simulink model "test_com_SensorFusion_SF_D4_slip_GPS"  (R2019b)
settings: Solver=FixedStepDiscrete  StartTime=0  StopTime=stop  FixedStep=0.001  RelTol=1e-3
undefined symbols (not defined in the file or in its folder): BxTM, ByTM, CxTM, CyTM, g, gamma_stat_front, gamma_stat_rear, gearbox_ratio, l_F, l_R, m_sprung, m_unsprung_quarter, mag_calib_front_center, mag_calib_front_compmatrix, mag_calib_rear_center, mag_calib_rear_compmatrix, should_be_in_theSensorFusion, switch_VelYcalculation_pSF, testStart_VelX_pSF, testVelY_pSF, tire_r_dyn, track_angle_front, track_width_front, track_width_rear, v2o_x, wheel_kinematics_breakpoints, wheel_kinematics_FL_data, wheel_kinematics_FR_data, wheelbase, x9DFrontX, x9DFrontY, x9DRearX, x9DRearY
libraries: SignalProcessingSensorFusionLib x30, simulink x6
(part 8 of 9)

== matlab function test_com_SensorFusion_SF_D4_slip_GPS/Subsystem14/SensorFusion_D4/SF_LaKl_GPS ==
  data: x9DFront input Bus: control_9D; VehicleState output Bus: control_VehicleState; x9DRear input Bus: control_9D; v2o input Bus: control_Velocity; WheelSpeeds input; WheelSpeeds_Sq input; RockerAngle input; RockerAngle_Sq input; dt input; kalman_running output; tire_r_dyn parameter; GPS input
function [VehicleState,kalman_running]  = fcn(x9DFront, x9DRear, v2o, WheelSpeeds, WheelSpeeds_Sq, RockerAngle, RockerAngle_Sq, dt, tire_r_dyn, GPS)
%% SAE is the used KOS, global not local on the car -> trafo of measurements in global KOS necessary
persistent state P

persistent standstill_counter
persistent bias_measurements 
persistent P_bias

persistent YawAngle_Front_old YawAngle_Rear_old v2o_VelX_old


num_states= 7;
num_measurements=5;


% copied from E10 SF .. might work
YawAngle_measurement=single(0);
R_YawAngle=1000;


% state   =   (1) PosX
%             (2) PosY
%             (3) PosZ
%             (4) VelX
%             (5) VelY
%             (6) VelZ
%             (7) YawAngle
%             (8)YawRate
% %             (9)WheelVelocity_FL
% %             (10)WheelVelocity_FR
% %             (11)WheelVelocity_RL
% %             (12)WheelVelocity_RR
     

% Actually used measurements:
%               (1) VelX
%               (2) VelY
%               (3) AccX front
%               (4) AccY front
%               (5) AccZ front
%               (6) YawAngle_Front
%               (7) YawRate_Front
%               (8) wheelvelocity_FL
%               (9) wheelvelocity_FR
%               (10) wheelvelocity_RL
%               (11)wheelvelocity_RR



if isempty(P)
    
    P_bias=single(eye(num_measurements));%*0.01);
    standstill_counter=0;
    bias_measurements=single(zeros(num_measurements,1));
    

    state = single(zeros(num_states,1));
    P = single(eye(num_states, num_states));%*0.1);
    
    YawAngle_Front_old=single(0);
    YawAngle_Rear_old=single(0);
    v2o_VelX_old=single(0);
    
end




%% Readability

PosX=       state(1);
PosY=       state(2);
PosZ=       state(3);
VelX=       state(4);
VelY=       state(5);
VelZ=       state(6);
YawAngle=   state(7);
%YawRate=    state(8);
% Wheelvel_FL= state(9);
% Wheelvel_FR= state(10);
% Wheelvel_RL= state(11);
% Wheelvel_RR= state(12);

AccX = x9DFront.AccX;
AccY = x9DFront.AccY;
AccZ = x9DFront.AccZ;
YawRate = x9DFront.YawRate;
GPS_Long = (GPS.GPS_Longitude-8.5);%*100000;
GPS_Lat = (GPS.GPS_Latitude-49.30);%*100000;


    measurements= [
% v2o.VelX            % (1)   v2o Sensor x velocity
% v2o.VelY            % (2)   v2o Sensor y velocity
% v2o.SlipAngle       % (3)   v2o Sensor Slipangle
% x9DFront.AccX       % (4)   IMU Front  x acceleration
% x9DFront.AccY       % (5)   IMU Front  y acceleration
% x9DFront.AccZ       % (6)   IMU Front  z acceleration
% x9DFront.RollRate   % (7)   IMU Front  RollRate
% x9DFront.PitchRate  % (8)   IMU Front  PitchRate
% x9DFront.YawRate    % (9)   IMU Front  YawRate
% x9DFront.MagX       % (10)  IMU Front  RollAngle
% x9DFront.MagY       % (11)  IMU Front  PitchAngle
% x9DFront.MagZ       % (12)  IMU Front  YawAngle
% x9DRear.AccX        % (13)  IMU Rear   x acceleration
% x9DRear.AccY        % (14)  IMU Rear   y acceleration
% x9DRear.AccZ        % (15)  IMU Rear   z acceleration
% x9DRear.RollRate    % (16)  IMU Rear   RollRate
% x9DRear.PitchRate   % (17)  IMU Rear   PitchRate
% x9DRear.YawRate     % (18)  IMU Rear   YawRate
% x9DRear.MagX        % (19)  IMU Rear   RollAngle
% x9DRear.MagY        % (20)  IMU Rear   PitchAngle
% x9DRear.MagZ        % (21)  IMU Rear   YawRAngle
% WheelSpeeds(1)      % (22)  wheelspeed  FL
% WheelSpeeds(2)      % (23)  wheelspeed  FR
% WheelSpeeds(3)      % (24)  wheelspeed  RL
% WheelSpeeds(4)      % (25)  wheelspeed  RR
% RockerAngle(1)      % (26)  Rockerangle FL
% RockerAngle(2)      % (27)  Rockerangle FR
% RockerAngle(3)      % (28)  Rockerangle RL
% RockerAngle(4)      % (29)  Rockerangle RR
GPS_Long;
GPS_Lat;
v2o.VelX              % (1)  v2o Sensor  x velocity
v2o.VelY              % (2)  v2o Sensor  y velocity
YawAngle_measurement
%x9DFront.AccX         % (3)  IMU Front Acceleration X
%x9DFront.AccY         % (4)  IMU Front Acceleration Y
%x9DFront.AccZ         % (5)  IMU Front Acceleration Z
%v2o.SlipAngle          % (6)  v20 Front   YawAngle
%x9DFront.YawRate      % (7)  IMU Front   YawRate
% WheelSpeeds(1)        % (8)  wheelspeed  FL
% WheelSpeeds(2)        % (9)  wheelspeed  FR
% WheelSpeeds(3)        % (10) wheelspeed  RL
% WheelSpeeds(4)        % (11) wheelspeed  RR
];



measurements_Sq= [
% v2o.VelX_Sq            % (1)   v2o Sensor x velocity        Signal Quality
% v2o.VelY_Sq            % (2)   v2o Sensor y velocity        Signal Quality
% v2o.SlipAngle_Sq       % (3)   v2o Sensor Slipangle         Signal Quality
% x9DFront.AccX_Sq       % (4)   IMU Front  x acceleration    Signal Quality
% x9DFront.AccY_Sq       % (5)   IMU Front  y acceleration    Signal Quality
% x9DFront.AccZ_Sq       % (6)   IMU Front  z acceleration    Signal Quality
% x9DFront.RollRate_Sq   % (7)   IMU Front  RollRate          Signal Quality
% x9DFront.PitchRate_Sq  % (8)   IMU Front  PitchRate         Signal Quality
% x9DFront.YawRate_Sq    % (9)   IMU Front  YawRate           Signal Quality
% 0                      % (10)  IMU Front  RollAngle         Signal Quality
% 0                      % (11)  IMU Front  PitchAngle        Signal Quality
% 0                      % (12)  IMU Front  YawAngle          Signal Quality
% x9DRear.AccX_Sq        % (13)  IMU Rear   x acceleration    Signal Quality
% x9DRear.AccY_Sq        % (14)  IMU Rear   y acceleration    Signal Quality
% x9DRear.AccZ_Sq        % (15)  IMU Rear   z acceleration    Signal Quality
% x9DRear.RollRate_Sq    % (16)  IMU Rear   RollRate          Signal Quality
% x9DRear.PitchRate_Sq   % (17)  IMU Rear   PitchRate         Signal Quality
% x9DRear.YawRate_Sq     % (18)  IMU Rear   YawRate           Signal Quality
% 0                      % (19)  IMU Rear   RollAngle         Signal Quality
% 0                      % (20)  IMU Rear   PitchAngle        Signal Quality
% 0                      % (21)  IMU Rear   YawAngle          Signal Quality
% WheelSpeeds_Sq(1)      % (22)  wheelspeed FL                Signal Quality
% WheelSpeeds_Sq(2)      % (23)  wheelspeed FR                Signal Quality
% WheelSpeeds_Sq(3)      % (24)  wheelspeed RL                Signal Quality
% WheelSpeeds_Sq(4)      % (25)  wheelspeed RR                Signal Quality
% RockerAngle_Sq(1)      % (26)  RockerangleFL                Signal Quality
% RockerAngle_Sq(2)      % (27)  RockerangleFR                Signal Quality
% RockerAngle_Sq(3)      % (28)  RockerangleRL                Signal Quality
% RockerAngle_Sq(4)      % (29)  RockerangleRR                Signal Quality
0
0
v2o.VelX_Sq            % (1)   v2o Sensor x velocity         Signal Quality
v2o.VelY_Sq            % (2)   v2o Sensor y velocity         Signal Quality
0
%x9DFront.AccX_Sq       % (3)  IMU Front Acceleration X       Siganl Quality
%x9DFront.AccY_Sq       % (4)  IMU Front Acceleration Y       Signal Quality
%x9DFront.AccZ_Sq       % (5)  IMU Front Acceleration Z       Signal Quality
%0 %v2o.SlipAngle_Sq        % (6)  V2O Front  YawAngle            Signal Quality
%x9DFront.YawRate_Sq    % (7)  IMU Front  YawRate             Signal Quality
% WheelSpeeds_Sq(1)      % (8)  wheelspeed  FL                 Signal Quality
% WheelSpeeds_Sq(2)      % (9)  wheelspeed  FR                 Signal Quality
% WheelSpeeds_Sq(3)      % (10)  wheelspeed  RL                 Signal Quality
% WheelSpeeds_Sq(4)      % (11)  wheelspeed  RR                 Signal Quality
];




%Correction of the sensor inputs with the estimated biases
% nb == no bias
measurements_nb=    measurements-bias_measurements;
WheelSpeeds_nb=     single(zeros(4,1));
% RockerAngle_nb=     single(zeros(4,1));
    
% v2o_VelX_nb=                measurements_nb(1);
% v2o_VelY_nb=                measurements_nb(2);
% v2o_SlipAngle_nb=           measurements_nb(3);
% x9D_Front_AccX_nb=          measurements_nb(4);
% x9D_Front_AccY_nb=          measurements_nb(5);
% x9D_Front_AccZ_nb=          measurements_nb(6); 
% x9D_Front_RollRate_nb=      measurements_nb(7);
% x9D_Front_PitchRate_nb=     measurements_nb(8);
% x9D_Front_YawRate_nb=       measurements_nb(9);
% x9D_Front_RollAngle_nb=     measurements_nb(10);
% x9D_Front_PitchAngle_nb=    measurements_nb(11);
% x9D_Front_YawAngle_nb=      measurements_nb(12);
% x9D_Rear_AccX_nb=           measurements_nb(13);
% x9D_Rear_AccY_nb=           measurements_nb(14);
% x9D_Rear_AccZ_nb=           measurements_nb(15); 
% x9D_Rear_RollRate_nb=       measurements_nb(16);
% x9D_Rear_PitchRate_nb=      measurements_nb(17);
% x9D_Rear_YawRate_nb=        measurements_nb(18);
% x9D_Rear_RollAngle_nb=      measurements_nb(19);
% x9D_Rear_PitchAngle_nb=     measurements_nb(20);
% x9D_Rear_YawAngle_nb=       measurements_nb(21);
% WheelSpeeds_nb(1)=          measurements_nb(22);
% WheelSpeeds_nb(2)=          measurements_nb(23);
% WheelSpeeds_nb(3)=          measurements_nb(24);
% WheelSpeeds_nb(4)=          measurements_nb(25);
% RockerAngle_nb(1)=          measurements_nb(26);
% RockerAngle_nb(2)=          measurements_nb(27);
% RockerAngle_nb(3)=          measurements_nb(28);
% RockerAngle_nb(4)=          measurements_nb(29);
GPS_Long_nb=                measurements_nb(1);
GPS_Lat_nb=                 measurements_nb(2);
v2o_VelX_nb=                measurements_nb(3);
v2o_VelY_nb=                measurements_nb(4);
YawAngle_nb=                measurements_nb(5);
%v2o_Slip_nb=                measurements_nb(5);
%x9D_Front_AccX_nb=          measurements_nb(3);
%x9D_Front_AccY_nb=          measurements_nb(4);
%x9D_Front_AccZ_nb=          measurements_nb(5);
%x9D_Front_YawAngle_nb=      measurements_nb(3);
%x9D_Front_YawRate_nb=       measurements_nb(7);
% WheelSpeeds_nb(1)=          measurements_nb(8);
% WheelSpeeds_nb(2)=          measurements_nb(9);
% WheelSpeeds_nb(3)=          measurements_nb(10);
% WheelSpeeds_nb(4)=          measurements_nb(11);




% system dynamics (nonlinear)
    
%     
% x(k+1)=f(x(k))=[ PosX + cos(YawAngle)VelX + sin(YawAngle)VelY
%                  PosY - sin(YawAngle)VelX + cos(YawAngle)VelY
%                  PosZ + VelZ
%                  VelX+dt*(AccX+VelY*YawRate)      %%%VelX + cos(YawAngle)AccX - sin(YawAngle)YawRate*VelX + sin(YawAngle)AccY + cos(YawAngle)YawRate*VelY
%                  VelY+dt*(AccY-VelX*YawRate)      %%%VelY - sin(YawAngle)AccX - cos(YawAngle)YawRate*VelX + cos(YawAngle)AccY - sin(YawAngle)YawRate*VelY
%                  VelZ + AccZ
%                  YawAngle + YawRate
% %                  Wheelspeeds?
% %                  Wheelspeeds?
% %                  Wheelspeeds?
% %                  Wheelspeeds?]


    %system dynamics Jacobi matrix (linearized)
    
%  PosX PosY PosZ              VelX        VelY       VelZ                    YawAngle                            
% J=[1    0    0    cos(YawAngle)*dt    sin(YawAngle)*dt    0    -sin(YawAngle)*VelX*dt+cos(YawAngle)*VelY*dt      %PosX
%    0    1    0    -sin(YawAngle)*dt  cos(YawAngle)*dt     0    -cos(YawAngle)*VelX*dt-sin(YawAngle)*VelY*dt       %PosY
%    0    0    1                 0                  0       dt        0                                          %PosZ
%    0    0    0    1-sin(YawAngle)*YawRate*dt     cos(YawAngle)*YawRate*dt   0   -sin(YawAngle)*AccX*dt+sin(YawAngle)*YawRate*VelX*dt+cos(YawAngle)*AccY*dt-sin(YawAngle)*YawRate*VelY*dt %VelX
%    0    0    0     -cos(YawAngle)*YawRate*dt   1-sin(YawAngle)*YawRate*dt  0   -cos(YawAngle)*AccX*dt+sin(YawAngle)*YawRate*VelX*dt-sin(YawAngle)*AccY*dt-cos(YawAngle)*YawRate*VelY*dt %VelY
%    0    0    0                 0                  0                1+AccZ*dt                 0    %VelZ
%    0    0    0                 0                  0                   0                      1];%YawAngle

J=[1    0   0   cos(YawAngle)*dt    sin(YawAngle)*dt   0   -sin(YawAngle)*VelX*dt+cos(YawAngle)*VelY*dt      %PosX
   0    1   0    -sin(YawAngle)*dt  cos(YawAngle)*dt  0   -cos(YawAngle)*VelX*dt-sin(YawAngle)*VelY*dt       %PosY
   0    0    1   0   0   0   0
   0    0   0    1     YawRate*dt   0 0%VelX
   0    0   0     YawRate*dt   1   0 0%VelY
   0    0   0            0   0  0  1
   0    0   0               0                   0       0               1];%YawAngle

% J=[1    0    0    0    0      %PosX
%    0    1    0    0    0       %PosY                                        %PosZ
%    0    0    1     YawRate*dt    0 %VelX
%    0    0    YawRate*dt   1  0 %VelY   %VelZ
%    0    0               0                  0                              1];%YawAngle
% 
% 



%Process noise Covariance matrix
                            
  %This matrix describes the process noise.
  %It determines how much the predicted
  %state is taken into account for the actual
  %state, the higher the values, the less the
  %predicion is taken into account for this state.
                                    
Q=diag([0.001   %(1) PosX
        0.001   %(2) PosY
        0.1     %(3) PosZ
        0.1    %(4) VelX
        0.1    %(5) VelY
        0.1     %(6) VelZ
        0.0001 ]);   %(7) YawAngle E-9
%         0.2 %(10) YawRate
%         0.1   %(11) Wvel_FL
%         0.1   %(12) Wvel_FR
%         0.1   %(13) Wvel_RL
%         0.1]);%(14) Wvel_RR


    
    
%Measurement noise Covariance matrix

 %This matrix determines how much the
 %measurments are taken into account. The
 %higher, the less they are taken into account.

% R=diag([0.1  %(1) VelX
%         0.1  %(2) VelY
%         0.1   %(3) YawAngle_Front
%         0.10  %(4) YawRate_Front
%         1    %(5) YawAngle_Rear
%         1    %(6) YawRate_Rear
%         1    %(7) wheelvelocity_FL
%         1    %(8) wheelvelocity_FR
%         1    %(9) wheelvelocity_RL
%         1]); %(10)wheelvelocity_RR
    
    
R=diag([10
        10
        0.1 %(1) VelX
        0.1   %(2) VelY
        10]); % (3) YawAngle_Front
%         0.1    % (3) Acceleration x
%         0.1    % (4) Acceleration y
%         0.1    % (5) Acceleration z
%         0.1    %(4) YawRate_Front         
%         0.3     %(5) wheelvelocity_FL
%         0.3     %(6) wheelvelocity_FR
%         0.3     %(7) wheelvelocity_RL
%         0.3]);  %(8)wheelvelocity_RR
 
    

     %Measurement matrix
     
%      %PosX  %PosY %PosZ  %VelX  %VelY  %VelZ %AccX %AccY %AccZ %YawAn %YawR %Wvel_FL %Wvel_FR %Wvel_RL %Wvel_RR
% H= [ 0      0     0      cos(YawAngle)      -sin(YawAngle)      0     -sin(YawAngle)*VelX-cos(YawAngle)*VelY             %VelX
%      0      0     0      sin(YawAngle)      cos(YawAngle)      0     cos(YawAngle)*VelX-sin(YawAngle)*VelY             %VelY
%      0      0     0      0      0      0     1];             %YawAngle_Front
 
 
 H=[ 1      0      0      0      0      0     0
     0      1      0      0      0      0     0
     0      0      0      1      0      0     0        %VelX
     0      0      0      0      1      0     0         %VelY
     0      0      0      0      0      0     1 ];           %YawAngle_Front
 
%      0      0     0      0      0      0     0     1     0     0      0        %Acceleration X
%      0      0     0      0      0      0     0     0     1     0      0        %Acceleration Y
%      0      0     0      0      0      0     0     0     0     0      1        %Acceleration Z
%      0      0     0      0      0      0     0     0     0     0      1];      %YawRate_Front
%      0      0     0      0      0      0     0     0     0     0      0     
%      0      0     0      0      0      0     0     0     0     0      0     
%      0      0     0      0      0      0     0     0     0     0      0];  %wheelvelocity_RR
     
     
     
avgWheelSpeed=mean(abs(WheelSpeeds));


if (avgWheelSpeed < 0.02 )
        vehicle_is_driving=false;
        standstill_counter=standstill_counter+1;
else
        vehicle_is_driving=true;
        standstill_counter=0;
end


bias_measurement_running=false;
kalman_running=false;
vehicle_is_driving=true;
if (~vehicle_is_driving)
    
    

    if standstill_counter*dt>2 && standstill_counter*dt<10
    bias_measurement_running=true;    
    kill_matrix_bias=zeros(num_measurements,num_measurements);
        for i=1:num_measurements
            if measurements_Sq(i)<4
                kill_matrix_bias(i,i)=1;
            end
        end
        H_bias=kill_matrix_bias;
        R_bias=eye(num_measurements)*0.01;  % Sinnvolle Werte?
        I_bias=eye(num_measurements);
        
        Z_bias = kill_matrix_bias*measurements;
        w_bias = Z_bias-(H_bias*bias_measurements);
        K_bias = (P_bias*H_bias')/(H_bias*P_bias*H_bias.'+R_bias);  
        bias_measurements = bias_measurements+K_bias*w_bias;
        P_bias = (I_bias-K_bias*H_bias)*P_bias;
    end

    
    
    
    
else 
        
    kalman_running=true;
    
    
%% Prediction step
% should be in the same coordinate system -> global or body-attached
% prediction of the state
    x1 =[ PosX+cos(YawAngle)*dt*VelX+sin(YawAngle)*VelY*dt;  %(1) PosX
             PosY-sin(YawAngle)*VelX*dt+dt*VelY*cos(YawAngle);  %(2) PosY
            PosZ + VelZ*dt                       %(3) PosZ
             VelX+dt*(AccX+VelY*YawRate);               %%%%VelX+cos(YawAngle)*AccX*dt-sin(YawAngle)*YawRate*VelX*dt+sin(YawAngle)*AccY+cos(YawAngle)*YawRate*VelY*dt                       %(4) VelX
             VelY+dt*(AccY-VelX*YawRate);               %%%%%VelY-sin(YawAngle)*AccX*dt-cos(YawAngle)*YawRate*VelX*dt+cos(YawAngle)*AccY-sin(YawAngle)*YawRate*VelY*dt                     %(5) VelY
            VelZ+AccZ*dt                     %(6) VelZ
             YawAngle+dt*YawRate ];       %(10) YawAngle
%             YawRate                   %(11) YawRate
%              Wheelvel_FL                %(12) Wheel velocity front left
%              Wheelvel_FR                %(13) Wheel velocity front right 
%              Wheelvel_RL                %(14) Wheel velocity rear left
%              Wheelvel_RR];              %(15) Wheel velocity rear right
           
% prediction of the covariance matrix
     P = J*P*J' + Q;
    
  
end 



%% Update step

%Verwendete Messung für v2o VelX
use_v2o_VelX=0;
v2o_VelX_used_measurement=single(0);
if (v2o.VelX_Sq<4) && (v2o.VelY_Sq<4) && abs(v2o_VelX_nb-v2o_VelX_old) < 2
    
    v2o_VelX_used_measurement=v2o_VelX_nb;

    use_v2o_VelX=1;

end

if(v2o_VelX_old~=v2o_VelX_nb)
    v2o_VelX_old=v2o_VelX_nb;
end


%Verwendete Messung für v2o VelY

use_v2o_VelY=0;
v2o_VelY_used_measurement=single(0);



%Verwendete Messung für 9DFront YawAngle

use_9DFront_YawAngle=0;
%x9DFront_YawAngle_used_measurement=single(0);
% x9DFront_YawAngle_used_measurement= x9DFront.MagZ;
% if (x9DFront.YawRate_Sq<4)
%     
%     x9DFront_YawAngle_used_measurement=x9D_Front_YawAngle_nb*(pi/180);
%     
%     use_9DFront_YawAngle=1;
%     
% end


%Verwendete Messung für 9DFront YawRate

use_9DFront_YawRate=0;
x9DFront_YawRate_used_measurement=single(0);

% if (x9DFront.YawRate_Sq<4)
%     
%     x9DFront_YawRate_used_measurement=x9D_Front_YawRate_nb;
%     
%     use_9DFront_YawRate=1;
%     
% end

%Verwendete Messung für 9DRear YawAngle
% 
% use_9DRear_YawAngle=0;
% x9DRear_YawAngle_used_measurement=single(0);
% 
% if (x9DRear.YawRate_Sq<4)
%     
%     x9DRear_YawAngle_used_measurement=x9D_Rear_YawAngle_nb*(pi/180);
%     
%     use_9DRear_YawAngle=1;
%     
% end
% 
% %Verwendete Messung für 9DRear YawRate
% 
% use_9DRear_YawRate=0;
% x9DRear_YawRate_used_measurement=single(0);
% 
% if (x9DRear.YawRate_Sq<4)
%     
%     x9DRear_YawRate_used_measurement=x9D_Rear_YawRate_nb;
%     
%     use_9DRear_YawRate=1;
%     
% end

% 
% % Limitierung der YawAngle auf -pi - pi wird aufgehoben
if(YawAngle_Front_old-YawAngle_nb < -180)
YawAngle_nb = YawAngle_nb - round(abs(YawAngle_Front_old-YawAngle_nb)/(2*180))*2*180;
elseif(YawAngle_Front_old-YawAngle_nb > 180)
YawAngle_nb = YawAngle_nb + round(abs(YawAngle_Front_old-YawAngle_nb)/(2*180))*2*180;
end

% if(YawAngle_Rear_old-x9D_Rear_YawAngle_nb < -180)
% x9D_Rear_YawAngle_nb = x9D_Rear_YawAngle_nb - round(abs(YawAngle_Rear_old-x9D_Rear_YawAngle_nb)/(2*180))*2*180;
% elseif(YawAngle_Rear_old-x9D_Rear_YawAngle_nb > 180)
% x9D_Rear_YawAngle_nb = x9D_Rear_YawAngle_nb + round(abs(YawAngle_Rear_old-x9D_Rear_YawAngle_nb)/(2*180))*2*180;
% end

%YawAngle_Front_old=x9D_Front_YawAngle_nb;
% YawAngle_Rear_old=x9D_Rear_YawAngle_nb;




%Verwendete Messung für wheelvelocity FL
use_wheelvelocity_FL=0;
wheelvelocity_FL_used_measurement=single(0);

if WheelSpeeds_Sq(1)<3
    
    wheelvelocity_FL_used_measurement=WheelSpeeds_nb(1)*tire_r_dyn;
    
    use_wheelvelocity_FL=1;

end


%Verwendete Messung für wheelvelocity FR
use_wheelvelocity_FR=0;
wheelvelocity_FR_used_measurement=single(0);

if WheelSpeeds_Sq(2)<3
    
    wheelvelocity_FR_used_measurement=WheelSpeeds_nb(2)*tire_r_dyn;
    
    use_wheelvelocity_FR=1;

end



%Verwendete Messung für wheelvelocity RL
use_wheelvelocity_RL=0;
wheelvelocity_RL_used_measurement=single(0);

if WheelSpeeds_Sq(3)<3
    
    wheelvelocity_RL_used_measurement=WheelSpeeds_nb(3)*tire_r_dyn;
    
    use_wheelvelocity_RL=1;

end



%Verwendete Messung für wheelvelocity RR
use_wheelvelocity_RR=0;
wheelvelocity_RR_used_measurement=single(0);

if WheelSpeeds_Sq(4)<3
    
    wheelvelocity_RR_used_measurement=WheelSpeeds_nb(4)*tire_r_dyn;
    
    use_wheelvelocity_RR=1;

end



% kill_measurements=[ use_v2o_VelX
%                     use_v2o_VelY
%                     use_9DFront_YawAngle
%                     use_9DFront_YawRate
%                     use_wheelvelocity_FL
%                     use_wheelvelocity_FR
%                     use_wheelvelocity_RL
%                     use_wheelvelocity_RR];

%new z with transformation
% z = [cos(YawAngle)*v2o_VelX_nb-sin(YawAngle)*v2o_VelY_nb;...
%     sin(YawAngle)*v2o_VelX_nb+cos(YawAngle)*v2o_VelY_nb;...
%     x9D_Front_YawAngle_nb];

z  = [GPS_Long_nb;...
    GPS_Lat_nb;...
    v2o_VelX_nb;...
    v2o_VelY_nb;...
    YawAngle_nb];%single(0)


% z=[ v2o_VelX_used_measurement
%     v2o_VelY_used_measurement
% %     x9DFront.AccX
% %     x9DFront.AccY
% %     x9DFront.AccZ
%     x9DFront_YawAngle_used_measurement];
%     x9DFront_YawRate_used_measurement];
%     wheelvelocity_FL_used_measurement
%     wheelvelocity_FR_used_measurement
%     wheelvelocity_RL_used_measurement
%     wheelvelocity_RR_used_measurement];%.*kill_measurements;
                

z1=[x1(1);...
    x1(2);...
    x1(4);...
    x1(5);...
    x1(7)];




P12=P*H';                   %cross covariance
% K=P12*inv(H*P12+R);       %Kalman filter gain
% x=x1+K*(z-z1);            %state estimate
% P=P-K*P12';               %state covariance matrix


R=chol(H*P12+R);            %Cholesky factorization
U=P12/R;  %K=U/R'; Faster because of back substitution

state=x1+U*(R'\(z-z1));         %Back substitution to get state update
P=P-U*U';


% 
% I = eye(length(state));
% % H=diag(kill_measurements)*H;
% 
% % calculation of Kalman-Gain
% K = P*H'/(H*P*H'+R);
% 
% % update step to get x(k+1)=x(k)+K*(z-H*x(k))
% state=state+K*(z-H*state);
% 
% P=(I-K*H)*P;

% Plausibility check
if VelX<0
    VelX=single(0);
end

if ~vehicle_is_driving
    VelX=single(0); 
    VelY=single(0); 
    YawRate=single(0); 
end



VehicleState.PosX = PosX;
VehicleState.PosY = PosY;
VehicleState.VelX = VelX;
VehicleState.VelY = VelY;
VehicleState.YawAngle = YawAngle;
VehicleState.YawRate = YawRate;
VehicleState.YawAcc = single(0);
VehicleState.AccX = x9DFront.AccX;
VehicleState.AccY = x9DFront.AccY;
VehicleState.AccZ = single(0);
VehicleState.isDriving = vehicle_is_driving;





used_bias.VelX_bias=bias_measurements(3);
used_bias.VelY_bias=bias_measurements(4);
used_bias.YawAngle_9DFront_bias= bias_measurements(5);
used_bias.YawRate_9DFront_bias=single(0); %bias_measurements(4);
used_bias.YawAngle_9DRear_bias=single(0);
used_bias.YawRate_9DRear_bias=single(0);
used_bias.wheelvelocity_FL_bias=single(0); %bias_measurements(5);
used_bias.wheelvelocity_FR_bias=single(0); %bias_measurements(6);
used_bias.wheelvelocity_RL_bias=single(0); %bias_measurements(7);
used_bias.wheelvelocity_RR_bias=single(0); %bias_measurements(8);



used_measurements.VelX_measurement=z(3);
used_measurements.VelY_measurement=z(4);
used_measurements.YawAngle_9DFront_measurement=single(0); %z(3);


used_measurements.YawRate_9DFront_measurement=single(0); %z(4);
used_measurements.YawAngle_9DRear_measurement=single(0);
used_measurements.YawRate_9DRear_measurement=single(0);
used_measurements.wheelvelocity_FL_measurement=single(0); %z(5);
used_measurements.wheelvelocity_FR_measurement=single(0); %z(6);
used_measurements.wheelvelocity_RL_measurement=single(0); %z(7);
used_measurements.wheelvelocity_RR_measurement=single(0); %z(8);
end
%     
% VehicleState.PosX = single(0);
% VehicleState.PosY =single(0);
% VehicleState.VelX = single(0);
% VehicleState.VelY = single(0);
% VehicleState.YawAngle = single(0);
% VehicleState.YawRate = single(0);
% VehicleState.YawAcc = single(0);
% VehicleState.AccX = single(0);
% VehicleState.AccY = single(0);
% VehicleState.AccZ = single(0);
% VehicleState.isDriving = false;
% 
% 
% used_bias.VelX_bias=single(0);
% used_bias.VelY_bias=single(0);
% used_bias.YawAngle_9DFront_bias=single(0);
% used_bias.YawRate_9DFront_bias=single(0);
% used_bias.YawAngle_9DRear_bias=single(0);
% used_bias.YawRate_9DRear_bias=single(0);
% used_bias.wheelvelocity_FL_bias=single(0);
% used_bias.wheelvelocity_FR_bias=single(0);
% used_bias.wheelvelocity_RL_bias=single(0);
% used_bias.wheelvelocity_RR_bias=single(0);
% 
% 
% used_measurements.VelX_measurement=single(0);
% used_measurements.VelY_measurement=single(0);
% used_measurements.YawAngle_9DFront_measurement=single(0);
% used_measurements.YawRate_9DFront_measurement=single(0);
% used_measurements.YawAngle_9DRear_measurement=single(0);
% used_measurements.YawRate_9DRear_measurement=single(0);
% used_measurements.wheelvelocity_FL_measurement=single(0);
% used_measurements.wheelvelocity_FR_measurement=single(0);
% used_measurements.wheelvelocity_RL_measurement=single(0);
% used_measurements.wheelvelocity_RR_measurement=single(0);
% 
% bias_measurement_running=false;
% kalman_running=false;

== matlab function test_com_SensorFusion_SF_D4_slip_GPS/Subsystem14/SensorFusion_D4/MATLAB Function ==
  data: DriverDemand input; VehicleState output Bus: control_VehicleState; WheelSpeeds input; WheelAngle input; tire_r_dyn parameter; dt input single; l_F parameter; l_R parameter; TireSlipLong output; WheelVelocity output; WheelVelocity_old input single size=4; track_width_front parameter; track_width_rear parameter; wheelbase parameter
function [VehicleState, TireSlipLong, WheelVelocity] = Sensorless(DriverDemand, WheelSpeeds, WheelAngle, tire_r_dyn, dt, l_F, l_R, WheelVelocity_old, track_width_front, track_width_rear, wheelbase) 

% diese Funktion ist dafür da, wenn mit keinen Sensoren gefahren wird
% (Anfang der Saison)

WheelVelocity=tire_r_dyn*WheelSpeeds;
WheelVelocity_FL=WheelVelocity(1);
WheelVelocity_FR=WheelVelocity(2);
WheelVelocity_RL=WheelVelocity(3);
WheelVelocity_RR=WheelVelocity(4);

VelX_FL=(WheelVelocity(1))*cos(WheelAngle(1));
VelX_FR=WheelVelocity(2)*cos(WheelAngle(2)); %beim Beschleunigen HInterradantrieb, die Vorderen Räder sind stabiler, kein Schlupf
    
VelX=(VelX_FL+VelX_FR+WheelVelocity_RL+WheelVelocity_RR)/4;
AccX=single(0); 
TireSlipLong=[single(0); single(0); single(0); single(0)];

    WheelAcc_FL=(WheelVelocity_FL-WheelVelocity_old(1))/dt;
    WheelAcc_FR=(WheelVelocity_FR-WheelVelocity_old(2))/dt;
if DriverDemand>=0 
    VelX=(VelX_FL+VelX_FR)*0.5;
    AccX=(WheelAcc_FL+WheelAcc_FR)*0.5; 
    TireSlipLong=[single(0); single(0); -(WheelVelocity_RL-VelX)/max(abs(VelX), abs(WheelVelocity_RL)); -(WheelVelocity_RR-VelX)/max(abs(VelX), abs(WheelVelocity_RR))]; 
end    
   VelX_RL=(WheelVelocity(3));
    VelX_RR=WheelVelocity(4);
    WheelAcc_RL=(WheelVelocity_RL-WheelVelocity_old(3))/dt;
    WheelAcc_RR=(WheelVelocity_RR-WheelVelocity_old(4))/dt;   
if DriverDemand<0 % im Bremsfall, nur Vorderräder gebremst
    VelX=(VelX_RL+VelX_RR)*0.5;
    AccX=(WheelAcc_RL+WheelAcc_RR)*0.5;
    TireSlipLong=[(-(WheelVelocity_FL-VelX*cos(WheelAngle(1)))/max(abs(VelX*cos(WheelAngle(1))), abs(WheelVelocity_FL))); -((WheelVelocity_FR-VelX*cos(WheelAngle(2)))/max(abs(VelX*cos(WheelAngle(2))), abs(WheelVelocity_FR))); single(0); single(0)]; 
end  

%vel=YawRate*R einspurmodell

delta=(WheelAngle(1)+WheelAngle(2))*0.5;
r_y=single((wheelbase-VelX*0.03+0.0)*tan(sign(delta)*(pi*0.5)-0.2047*3.76*delta));

YawRate=(VelX*delta)/(l_F+l_R);
AccY=VelX*YawRate;
%VelY=(AccY-AccY_old)*dt;
%YawAcc=(YawRate-YawRate_old)/dt;



PosX=single(0);
PosY=single(0);
AccZ=single(0);
YawAngle=single(0);
YawAcc=single(0);
VelY=single(0);

VehicleState.PosX = PosX;
VehicleState.PosY = PosY;
VehicleState.VelX = VelX;
VehicleState.VelY = VelY;
VehicleState.YawAngle = YawAngle;
VehicleState.YawRate = YawRate;
VehicleState.YawAcc = YawAcc;
VehicleState.AccX = AccX;
VehicleState.AccY = AccY;
VehicleState.AccZ = AccZ;
VehicleState.isDriving = true;

vel = ([VelX; VelY; 0]);  
Rad = [l_F, l_F, -l_R, -l_R; -track_width_front/2, track_width_front/2, -track_width_rear/2, track_width_rear/2; 0, 0, 0, 0];  %Abstand cog zu rad mitte

       
omegaTilde = [0,-YawRate,0;...  % hier eigentlich noch Pitch und roll rate
                YawRate,0,0;...
                    0,0,0];

% velocity of tires 
velTire_FL = vel + omegaTilde * Rad(:,1);
velTire_FR = vel + omegaTilde * Rad(:,2);
velTire_RL = vel + omegaTilde * Rad(:,3);
velTire_RR = vel + omegaTilde * Rad(:,4);


%% Rotational matrices for Transformation from car coordinate system 
% into wheel coordinate systems
% rotMatrix_Front = [cos(delta),sin(delta),0; ... % hier eigentlich auch noch roll und pitch angle
%               -sin(delta),cos(delta),0;...
%               0,0,1];
WheelAngle_FL=WheelAngle(1);
WheelAngle_FR=WheelAngle(2);          
rotMatrix_FL = [cos(WheelAngle_FL),sin(WheelAngle_FL),0; ... % hier eigentlich auch noch roll und pitch angle
              -sin(WheelAngle_FL),cos(WheelAngle_FL),0;...
              0,0,1];
          
rotMatrix_FR = [cos(WheelAngle_FR),sin(WheelAngle_FR),0; ... % hier eigentlich auch noch roll und pitch angle
              -sin(WheelAngle_FR),cos(WheelAngle_FR),0;...
              0,0,1];
rotMatrix_Rear = [1,0,0; 0,1,0; 0,0,1];
 

% velocity of tires in tire coordinats (dieses Superpositionsprinzip ändert sich bei beta
% ungleich 0)
% wenn andere transformationsmatrix * durhch \ ersetzen
vel_help_FL = rotMatrix_FL * velTire_FL;
velX_FL = vel_help_FL(1);
velY_FL = vel_help_FL(2);
vel_help_FR = rotMatrix_FR* velTire_FR;
velX_FR = vel_help_FR(1);
velY_FR = vel_help_FR(2);
vel_help_RL = rotMatrix_Rear*velTire_RL;
velX_RL = vel_help_RL(1);
velY_RL = vel_help_RL(2);
vel_help_RR = rotMatrix_Rear*velTire_RR;
velX_RR = vel_help_RR(1);
velY_RR = vel_help_RR(2);

velX= single([velX_FL, velX_FR, velX_RL, velX_RR]);
velY= single([velY_FL, velY_FR, velY_RL, velY_RR]);



% relative velocities of wheels
velRelX_FL = WheelVelocity_FL - velX_FL;  %hier später die Zustände aus dem kalman filter für wheelspeeds
velRelX_FR = WheelVelocity_FR - velX_FR;
velRelX_RL = WheelVelocity_RL  - velX_RL;
velRelX_RR = WheelVelocity_RR  - velX_RR;


if(velX*ones(4,1) < 0.4) %TODO: Nachschauen, ob die Schwelle Probleme bereitet, oder ob diese höher oder tiefer gesetzt werden muss
    TireSlipLong = single([0, 0, 0, 0].');
end   
if(VelX< 0.4) %TODO: Nachschauen, ob die Schwelle Probleme bereitet, oder ob diese höher oder tiefer gesetzt werden muss
    TireSlipLong = single([0, 0, 0, 0].');
end 

for n=1:1:4
    if TireSlipLong(n) > 1
        TireSlipLong(n) = 1;
    elseif TireSlipLong(n) < -1
        TireSlipLong(n) = -1;
    end
end
end

== matlab function test_com_SensorFusion_SF_D4_slip_GPS/Subsystem14/SensorFusion_D4/MATLAB Function1 ==
  data: u input; y output
function y = fcn(u)
a=5;
b=14;
y=filter(b, a, u);
end

== matlab function test_com_SensorFusion_SF_D4_slip_GPS/Subsystem14/SensorFusion_D4/MATLAB Function2 ==
  data: WheelSpeeds input; WheelSpeeds_Sq input; WheelSpeeds_filtered output; dt input
function WheelSpeeds_filtered =  fc( WheelSpeeds, WheelSpeeds_Sq, dt)

persistent x P								

%Variablen für bias Messung
persistent standstill_counter
persistent bias_measurements 
persistent P_bias




%%
num_states=4;
num_measurements=4;
if isempty(P)
   
    
    
    %% bias Variablen Initialisierung
    P_bias=eye(num_measurements)*0.001;
    standstill_counter=0;
    bias_measurements=single(zeros(num_measurements,1));
    
    
    x = single(zeros(num_states,1));
    P = single(zeros(num_states, num_states));
	
  
end


%% Readability

    WheelVelocity_FL=x(1);
    WheelVelocity_FR=x(2);
    WheelVelocity_RL=x(3);
    WheelVelocity_RR=x(4);
    

    measurements= [
WheelSpeeds(1)      % (16)  wheelspeed  FL
WheelSpeeds(2)      % (17)  wheelspeed  FR
WheelSpeeds(3)      % (18)  wheelspeed  RL
WheelSpeeds(4)      % (19)  wheelspeed  RR
];

measurements_Sq= [
WheelSpeeds_Sq(1)      % (16)  wheelspeed  FL               Signal Quality
WheelSpeeds_Sq(2)      % (17)  wheelspeed  FR               Signal Quality
WheelSpeeds_Sq(3)      % (18)  wheelspeed  RL               Signal Quality
WheelSpeeds_Sq(4)      % (19)  wheelspeed  RR               Signal Quality
];


%Correction of the sensor inputs with the estimated biases
% nb == no bias
measurements_nb=    measurements-bias_measurements;
WheelSpeeds_nb=     single(zeros(4,1));

    

WheelSpeeds_nb(1)=      measurements_nb(1);
WheelSpeeds_nb(2)=      measurements_nb(2);
WheelSpeeds_nb(3)=      measurements_nb(3);
WheelSpeeds_nb(4)=      measurements_nb(4);


							  
									  																			 %% Preparing WheelSpeeds


% Durchschnittliche Radgeschwindigkeiten ermitteln
avgWheelVelocity = mean(WheelSpeeds);








%% Prediction 

if(avgWheelVelocity < 0.01 )
        vehicle_is_driving=false;
        standstill_counter=standstill_counter+1;
    else
        vehicle_is_driving=true;
        standstill_counter=0;
end


if ~vehicle_is_driving
    
    if standstill_counter*dt>0.5 && standstill_counter*dt<10
        
    kill_matrix_bias=zeros(num_measurements,num_measurements);
        for i=1:num_measurements
            if measurements_Sq(i)<4
                kill_matrix_bias(i,i)=1;
            end
        end
%         kill_matrix_bias=zeros(num_measurements,num_measurements);
        H_bias=kill_matrix_bias;
        R_bias=eye(num_measurements)*0.01;  % Sinnvolle Werte?
        I_bias=eye(num_measurements);
        
        Z_bias = kill_matrix_bias*measurements;
        w_bias = Z_bias-(H_bias*bias_measurements);
        K_bias = (P_bias*H_bias')/(H_bias*P_bias*H_bias.'+R_bias);  
        bias_measurements = bias_measurements+K_bias*w_bias;
        P_bias = (I_bias-K_bias*H_bias)*P_bias;
    end

    else % update the state only if the biases are currently not measured
        

   x=[  x(1);                                              % YawAcc;(18)  YawAcceleration of the Monocoque          
        x(2);                                              % wheelVelocity_FL;(19)  wheelspeed front left  wheel in rad         
        x(3);                                              %  wheelVelocity_FR;(20)  wheelspeed front right wheel in rad         
        x(4)];                                             % wheelVelocity_RL;(21)  wheelspeed rear  left  wheel in rad           ];                                              % wheelVelocity_RR;(22)  wheelspeed rear  right wheel in rad


    %Calculating a linearized A Matrix
          %PosX           VelX                AccX          PosY         VelY        AccY PosZ        VelZ          AccZ RollAngle  RollRate  RollAcc PitchAn PitchRate PitchAcc  YawAngle                                    YawRate YawAcc  19  20  21  22
    A=eye(4); 


    W = eye(num_states);

%     exp=single(0.4/((0.2*(x(5)-1)^2)+1)-2.4);%(0.4*(2^(-0.1*(x(5)-1)^2))-3.1);%-2.7*2^(-0.1*(x(5)-1)^2)-3.1*(-2^(-0.1*(x(5)-1)^2)+1) % This exponent is a value between -2.1 (if x(5)=2) and -4.5 (if x(5) is away from 2)
    % Covariance matrix of state noise
 Q = diag([
            1;       %WheelspeedFL;    % (19)  
            1;       %WheelspeedFR;    % (20)  
            1;       %WheedspeedRL;    % (21)  
            1]*0.001);  %WheelspeedRR;    % (22)   %dt
            

    % prediction calculation
    %x = x + dt*F*x; % + dt*B*u;          % statevector update
    %NO LINEAR EQUOTATION USED, THEREFORE ONLY THE LINEARIZED MATRIX A IS USED
    %TO UPDATE P

    P = A*P*A' + W*Q*W';                 % covariance matrix update
				   
end 


   

%% Measurement SF
% Measurement selection: With the help of the singal qualifiers it is
% determined which signal can be used as a measurement input for the kalman
% filter
%% Start der States
% Position X wird später bei uns von GPS gemessen noch kein info wie genau,
% bei Start wird Position auf null gesetzt
selection=[];

% WheelSpeeds (19) Front Left
if WheelSpeeds_Sq(1)<3
    WheelVelocity_FL_measurement=WheelSpeeds_nb(1);
    R_WheelVelocity_FL=0.0001;
    selection=[selection 1];
elseif WheelSpeeds_Sq(1)>4 && WheelSpeeds_Sq(2)<3 && WheelSpeeds_Sq(3)<3 && WheelSpeeds_nb(4)<3
    WheelVelocity_FL_measurement=(WheelSpeeds_nb(2)+WheelSpeeds_nb(3)+WheelSpeeds_nb(4))/3;%tire_r_dyn*
    R_WheelVelocity_FL=0.0001;
    selection=[selection 1];
else
    WheelVelocity_FL_measurement=single(0);
    R_WheelVelocity_FL=0.001;
end

% WheelSpeeds (20) Front Left
if WheelSpeeds_Sq(2)<3
    WheelVelocity_FR_measurement=WheelSpeeds_nb(2);
    R_WheelVelocity_FR=0.0001;
    selection=[selection 2];
elseif WheelSpeeds_Sq(2)>4 && WheelSpeeds_Sq(1)<3 && WheelSpeeds_Sq(3)<3 && WheelSpeeds_nb(4)<3
    WheelVelocity_FR_measurement= (WheelSpeeds_nb(1)+WheelSpeeds_nb(3)+WheelSpeeds_nb(4))/3;
    R_WheelVelocity_FR=0.0001;
    selection=[selection 2];
else
    WheelVelocity_FR_measurement=single(0);
    R_WheelVelocity_FR=0.1;
end

% WheelSpeeds (21) Front Left
if WheelSpeeds_Sq(3)<3
    WheelVelocity_RL_measurement=WheelSpeeds_nb(3);
    R_WheelVelocity_RL=0.0001;
    selection=[selection 3];
elseif WheelSpeeds_Sq(3)>4 && WheelSpeeds_Sq(1)<3 && WheelSpeeds_Sq(2)<3 && WheelSpeeds_nb(4)<3
    WheelVelocity_RL_measurement= (WheelSpeeds_nb(1)+WheelSpeeds_nb(2)+WheelSpeeds_nb(4))/3;
    R_WheelVelocity_RL=0.0001;
    selection=[selection 3];
else
    WheelVelocity_RL_measurement=single(0);
    R_WheelVelocity_RL=0.0001;
end
% WheelSpeeds (22) Front Left
if WheelSpeeds_Sq(4)<3
    WheelVelocity_RR_measurement=WheelSpeeds_nb(4);
    R_WheelVelocity_RR=0.0001;
    selection=[selection 4];
elseif WheelSpeeds_Sq(4)>4 && WheelSpeeds_Sq(1)<3 && WheelSpeeds_Sq(3)<3 && WheelSpeeds_nb(3)<3
    WheelVelocity_RR_measurement= (WheelSpeeds_nb(1)+WheelSpeeds_nb(3)+WheelSpeeds_nb(3))/3;
    R_WheelVelocity_RR=0.0001;
    selection=[selection 4];
else
  WheelVelocity_RR_measurement=single(0);
    R_WheelVelocity_RR=0.0001;
end



% Measured states
    
z1 = [ WheelVelocity_FL_measurement;     % WheelspeedFL (19)
      WheelVelocity_FR_measurement;     %WheelspeedFR  (20)
      WheelVelocity_RL_measurement;     %WheelspeedRL  (21)
      WheelVelocity_RR_measurement;   %WheelspeedRR (22)
    ];    
  

kill_matrix=zeros(length(z1),length(z1));
z=single(zeros(size(z1)));

for w=1:length(selection)
    z(selection(w))=z1(selection(w));    
    kill_matrix(selection(w),selection(w))=1.0;
end

h1=x;
h=kill_matrix*h1;

R = diag([
    1;                             % für die RH vgl mit RollANgle, PitchANgle und PosZ0.0
    1;
    1;
    1]);                    
H=eye(length(x));

% Correction equations
I = eye(length(x));
V = eye(length(z));

K_tmp = P*H'/(H*P*H'+V*R*V');

x = x + K_tmp*(z-h);
P = (I - K_tmp*H)*P;
WheelSpeeds_filtered=x;

== matlab function test_com_SensorFusion_SF_D4_slip_GPS/Subsystem14/SensorFusion_D4/MATLAB Function3 ==
  data: AccX input; AccX_filtered output
function AccX_filtered = fcn(AccX)
persistent x P

if isempty(P)
    P=single(0);
end

Q=0.001;
A=1;

    W = eye(1);


    P = A*P*A' + W*Q*W';                 % covariance matrix update
				   
end 

% Measured states
    
z = AccX;    
  
h=x;
R = 1;                  
H=eye(length(x));

% Correction equations
I = eye(length(x));
V = eye(length(z));

K_tmp = P*H'/(H*P*H'+V*R*V');

x = x + K_tmp*(z-h);
P = (I - K_tmp*H)*P;

x=AccX_filtered;

== matlab function test_com_SensorFusion_SF_D4_slip_GPS/Subsystem14/SensorFusion_D4/MATLAB Function4 ==
  data: AccX_Sq input; VD_diag_9Drear output; AccY_Sq input; AccZ_Sq input; YawRate_Sq input; PitchRate_Sq input; RollRate_Sq input
function VD_diag_9Drear = diag(AccX_Sq, AccY_Sq, AccZ_Sq, YawRate_Sq, PitchRate_Sq, RollRate_Sq)
bad_Sq_counter=single(0);
VD_diag_9Drear=0;
persistent timestep_counter_old
if isempty(timestep_counter_old)
    timestep_counter_old=0;
end


if AccX_Sq>4
    bad_Sq_counter=bad_Sq_counter+1;
end
if AccY_Sq>4
    bad_Sq_counter=bad_Sq_counter+1;
end
if AccZ_Sq>4
    bad_Sq_counter=bad_Sq_counter+1;
end
if YawRate_Sq>4
    bad_Sq_counter=bad_Sq_counter+1;
end
if RollRate_Sq>4
    bad_Sq_counter=bad_Sq_counter+1;
end
if PitchRate_Sq>4
    bad_Sq_counter=bad_Sq_counter+1;
end

if  bad_Sq_counter>3
    timestep_counter=timestep_counter_old+1;
else 
    timestep_counter=0;
end


if bad_Sq_counter>3 && timestep_counter >4
    VD_diag_9Drear=1;
end

timestep_counter_old=timestep_counter;

end

== matlab function test_com_SensorFusion_SF_D4_slip_GPS/Subsystem14/SensorFusion_D4/MATLAB Function5 ==
  data: VelX_Sq input; VD_diag_v2o output; VelY_Sq input; bad_Sq_counter output; timestep_counter output
function [VD_diag_v2o, bad_Sq_counter, timestep_counter] = diag(VelX_Sq, VelY_Sq)
bad_Sq_counter=single(0);
VD_diag_v2o=0;
persistent timestep_counter_old
if isempty(timestep_counter_old)
    timestep_counter_old=0;
end

if VelX_Sq>4
    bad_Sq_counter=bad_Sq_counter+1;
end
if VelY_Sq>4
    bad_Sq_counter=bad_Sq_counter+1;
end

if  bad_Sq_counter>1
    timestep_counter=timestep_counter_old+1;
else 
    timestep_counter=0;
end

if bad_Sq_counter>1 && timestep_counter >4
    VD_diag_v2o=1;
end

timestep_counter_old=timestep_counter;

end

== matlab function test_com_SensorFusion_SF_D4_slip_GPS/Subsystem14/SensorFusion_D4/MATLAB Function6 ==
  data: AccX_Sq input; VD_diag_9Dfront output; AccY_Sq input; AccZ_Sq input; YawRate_Sq input; PitchRate_Sq input; RollRate_Sq input
function VD_diag_9Dfront = diag(AccX_Sq, AccY_Sq, AccZ_Sq, YawRate_Sq, PitchRate_Sq, RollRate_Sq)
bad_Sq_counter=single(0);
VD_diag_9Dfront=0;
persistent timestep_counter_old
if isempty(timestep_counter_old)
    timestep_counter_old=0;
end


if AccX_Sq>4
    bad_Sq_counter=bad_Sq_counter+1;
end
if AccY_Sq>4
    bad_Sq_counter=bad_Sq_counter+1;
end
if AccZ_Sq>4
    bad_Sq_counter=bad_Sq_counter+1;
end
if YawRate_Sq>4
    bad_Sq_counter=bad_Sq_counter+1;
end
if RollRate_Sq>4
    bad_Sq_counter=bad_Sq_counter+1;
end
if PitchRate_Sq>4
    bad_Sq_counter=bad_Sq_counter+1;
end

if  bad_Sq_counter>3
    timestep_counter=timestep_counter_old+1;
else 
    timestep_counter=0;
end
if bad_Sq_counter>3 && timestep_counter >4
    VD_diag_9Dfront=1;
end

timestep_counter_old=timestep_counter;

end

== matlab function test_com_SensorFusion_SF_D4_slip_GPS/Subsystem14/SensorFusion_D4/MATLAB Function7 ==
  data: RockerAngle_FL_Sq input; VD_diag_RockerAngle output; RockerAngle_FR_Sq input; bad_Sq_counter output; timestep_counter output; RockerAngle_RL_Sq input; RockerAngle_RR_Sq input
function [VD_diag_RockerAngle, bad_Sq_counter, timestep_counter] = diag(RockerAngle_FL_Sq, RockerAngle_FR_Sq, RockerAngle_RL_Sq, RockerAngle_RR_Sq)
bad_Sq_counter=single(0);
VD_diag_RockerAngle=0;
persistent timestep_counter_old
if isempty(timestep_counter_old)
    timestep_counter_old=0;
end

if RockerAngle_FL_Sq>4
    bad_Sq_counter=bad_Sq_counter+1;
end
if RockerAngle_FR_Sq>4
    bad_Sq_counter=bad_Sq_counter+1;
end
if RockerAngle_RL_Sq>4
    bad_Sq_counter=bad_Sq_counter+1;
end
if RockerAngle_RR_Sq>4
    bad_Sq_counter=bad_Sq_counter+1;
end

if  bad_Sq_counter>1
    timestep_counter=timestep_counter_old+1;
else 
    timestep_counter=0;
end

if bad_Sq_counter>1 && timestep_counter >4
    VD_diag_RockerAngle=1;
end

timestep_counter_old=timestep_counter;

end

== matlab function test_com_SensorFusion_SF_D4_slip_GPS/Subsystem14/SensorFusion_D4/SiDes Testgelände ==
  data: measurements_nb input; easyYawRate_out output; x input; easyYawAngle_out output; easyPos_out output; wheelbase parameter; delta input; dt input; YawRateBySteer output
function [easyYawRate_out,easyYawAngle_out,easyPos_out,YawRateBySteer] = fcn(measurements_nb,x,wheelbase, delta,dt)

persistent easyPosX easyPosY easyYawAngle easyYawRate
persistent temp


if isempty(temp)
    temp=420;
       

    easyPosX =single(0);
    easyPosY =single(0);
    easyYawAngle =single(0);
    easyYawRate  =single(0);
end



PosX=x(1);
VelX=x(2);
AccX=x(3);
PosY=x(4);
VelY=x(5);
AccY=x(6);
PosZ=x(7);
VelZ=x(8);
AccZ=x(9);
RollAngle=x(10);
RollRate=x(11);
RollAcc=x(12);
PitchAngle=x(13);
PitchRate=x(14);
PitchAcc=x(15);
YawAngle=x(16);
YawRate=x(17);
YawAcc=x(18);
WheelSpeed_FL=x(19);
WheelSpeed_FR=x(20);
WheelSpeed_RL=x(21);
WheelSpeed_RR=x(22);

    WheelSpeeds_nb=     single(zeros(4,1));
    RockerAngle_nb=     single(zeros(4,1));

v2o_VelX_nb=            measurements_nb(1);
v2o_VelY_nb=            measurements_nb(2);
v2o_SlipAngle_nb=       measurements_nb(3);
x9D_Front_AccX_nb=      measurements_nb(4);
x9D_Front_AccY_nb=      measurements_nb(5);
x9D_Front_AccZ_nb=      measurements_nb(6);     %Gravitation berücksichtigen ???
x9D_Front_RollRate_nb=  measurements_nb(7);
x9D_Front_PitchRate_nb= measurements_nb(8);
x9D_Front_YawRate_nb=   measurements_nb(9);
x9D_Rear_AccX_nb=       measurements_nb(10);
x9D_Rear_AccY_nb=       measurements_nb(11);
x9D_Rear_AccZ_nb=       measurements_nb(12);    %Gravitation berücksichtigen ???
x9D_Rear_RollRate_nb=   measurements_nb(13);
x9D_Rear_PitchRate_nb=  measurements_nb(14);
x9D_Rear_YawRate_nb=    measurements_nb(15);
WheelSpeeds_nb(1)=      measurements_nb(16);
WheelSpeeds_nb(2)=      measurements_nb(17);
WheelSpeeds_nb(3)=      measurements_nb(18);
WheelSpeeds_nb(4)=      measurements_nb(19);
RockerAngle_nb(1)=      measurements_nb(20);
RockerAngle_nb(2)=      measurements_nb(21);
RockerAngle_nb(3)=      measurements_nb(22);
RockerAngle_nb(4)=      measurements_nb(23);

YawRate_factor=1.167;

easyYawRate=    (1/3)*(x9D_Front_YawRate_nb+x9D_Rear_YawRate_nb);
YawRateBySteer=(delta*VelX/wheelbase);
easyYawAngle=easyYawAngle+dt*easyYawRate;
easyPosX=easyPosX+cos(easyYawAngle*YawRate_factor)*dt*VelX-sin(easyYawAngle*YawRate_factor)*dt*VelY;
easyPosY=easyPosY+sin(easyYawAngle*YawRate_factor)*dt*VelX+cos(easyYawAngle*YawRate_factor)*dt*VelY;


easyYawRate_out=easyYawRate;
easyYawAngle_out=easyYawAngle;
easyPos_out=[easyPosX;easyPosY];

== matlab function test_com_SensorFusion_SF_D4_slip_GPS/Subsystem14/SensorFusion_D4/Sturzberechnung/MATLAB Function ==
  data: PosZ input; Camber_PosZ_front output; Camber_PosZ_rear output
function [Camber_PosZ_front, Camber_PosZ_rear] = fcn(PosZ)
Camber_PosZ_front=max(interp1([-25 -22.50 -20.00 -17.50 -15.00 -12.50 -10.00 -7.50 ...
    -5.00 -2.50 0.00 2.50 5.00 7.50 10.00 12.50 15.00 17.50 20.00 22.50 25.00 ], ...
    [-0.83 -0.74 -0.65 -0.56 -0.47 -0.39 -0.30 -0.23 -0.15 -0.07 0.00 0.07 0.14 0.20 ...
    0.27 0.33 0.39 0.44 0.50 0.55 0.60], PosZ,'spline'));
Camber_PosZ_rear=max(interp1([-25 -22.50 -20.00 -17.50 -15.00 -12.50 -10.00 -7.50 ...
    -5.00 -2.50 0.00 2.50 5.00 7.50 10.00 12.50 15.00 17.50 20.00 22.50 25.00],...
    [-0.64 -0.57 -0.50 -0.44 -0.37 -0.30 -0.24 -0.18 -0.12 -0.06 0.00 0.06 0.11 ...
    0.17 0.22 0.27 0.32 0.37 0.41 0.46 0.50], PosZ,'spline'));

end

== matlab function test_com_SensorFusion_SF_D4_slip_GPS/Subsystem14/SensorFusion_D4/Sturzberechnung/MATLAB Function1 ==
  data: Camber_RollAngle_front output; Camber_RollAngle_rear output; RollAngle input
function [Camber_RollAngle_front, Camber_RollAngle_rear]= fcn (RollAngle)
Camber_RollAngle_front=max(interp1([-1.50 -1.35 -1.20 -1.05 -0.90 -0.75 -0.60 -0.45 -0.30 -0.15 0.00 ...
0.15 0.30 0.45 0.60 0.75 0.90 1.05 1.20 1.35 1.50], ...
    [1.02 0.92 0.82 0.72 0.62 0.52 0.42 0.31 0.21 0.11 0.00 -0.11 -0.21 -0.32 -0.43 -0.53 -0.64 ...
-0.75 -0.86 -0.97 -1.08], RollAngle,'spline'));
Camber_RollAngle_rear=max(interp1([-1.50 -1.35 -1.20 -1.05 -0.90 -0.75 -0.60 -0.45 -0.30 -0.15 0.00 ...
0.15 0.30 0.45 0.60 0.75 0.90 1.05 1.20 1.35 1.50],...
    [1.11 1.00 0.89 0.78 0.67 0.56 0.45 0.34 0.23 0.11 0.00 -0.12 -0.23 -0.35 -0.46 -0.58 ...
-0.70 -0.81 -0.93 -1.05 -1.17], RollAngle,'spline'));
end
